simulink library "Tracked_ActiveSurveillance_Block"  (R2018b)
settings: Solver=VariableStepAuto  StartTime=0.0  StopTime=10.0  RelTol=1e-3
undefined symbols (not defined in the file): ac1dyn_alt0_ft, ac1dyn_lat0_rad, ac1dyn_lon0_rad, uas_tcas_dt_s, uas_tcas_trckd_altQuant_ft, uas_tcas_trckd_bearing_Breakpoints_deg, uas_tcas_trckd_bearing_Max_deg, uas_tcas_trckd_bearing_Sigma_deg, uas_tcas_trckd_FOR_elev_max_deg, uas_tcas_trckd_FOR_elev_min_deg, uas_tcas_trckd_probDetect, uas_tcas_trckd_psi_bias_rad, uas_tcas_trckd_psi_stddev_ft, uas_tcas_trckd_psidot_stddev_ftps, uas_tcas_trckd_randProbSeed, uas_tcas_trckd_reported_errorCovRBA, uas_tcas_trckd_rng_bias_ft, uas_tcas_trckd_rng_random_stddev_ft, uas_tcas_trckd_seed1, uas_tcas_trckd_seed2, uas_tcas_trckd_seed3, uas_tcas_trckd_seed4, uas_tcas_trckd_sns_max_front_range_ft, uas_tcas_trckd_sns_max_range_ft, uas_tcas_trckd_sns_max_rear_range_ft, uas_tcas_trckd_sns_max_side_range_ft, uas_tcas_trckd_tauThreshold_sec, uas_tcas_trckd_updateRate_sec
libraries: simulink x6, TSAA_Altitude_Error x1, dspmtrx3 x1
settings Model: Creator=BI28030  LastModifiedBy=BI28030

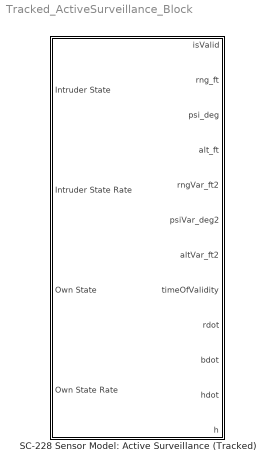
== system Tracked_ActiveSurveillance_Block ==
  SC-228 Sensor Model: Active Surveillance (Tracked) : Subsystem  mask(Tracked Surveillance: TCAS){dt_s=uas_tcas_dt_s, lat0_rad=ac1dyn_lat0_rad, lon0_rad=ac1dyn_lon0_rad, alt0_ft=ac1dyn_alt0_ft, sns_max_range_ft=uas_tcas_trckd_sns_max_range_ft, rng_random_stddev_ft=uas_tcas_trckd_rng_random_stddev_ft, rng_bias_ft=uas_tcas_trckd_rng_bias_ft, rng_tau_s=0, seed1=uas_tcas_trckd_seed1, bearing_Max_deg=uas_tcas_trckd_bearing_Max_deg, bearing_Sigma_deg=uas_tcas_trckd_bearing_Sigma_deg, bearing_Breakpoints_deg=uas_tcas_trckd_bearing_Breakpoints_deg, seed2=uas_tcas_trckd_seed2, seed3=uas_tcas_trckd_seed3, seed4=uas_tcas_trckd_seed4, altQuant_ft=uas_tcas_trckd_altQuant_ft, covRBA=uas_tcas_trckd_reported_errorCovRBA, sns_max_front_range_ft=uas_tcas_trckd_sns_max_front_range_ft, sns_max_side_range_ft=uas_tcas_trckd_sns_max_side_range_ft, sns_max_rear_range_ft=uas_tcas_trckd_sns_max_rear_range_ft, probDetect=uas_tcas_trckd_probDetect, FOR_elev_max_deg=uas_tcas_trckd_FOR_elev_max_deg, FOR_elev_min_deg=uas_tcas_trckd_FOR_elev_min_deg, randProbSeed=uas_tcas_trckd_randProbSeed, tauThreshold_sec=uas_tcas_trckd_tauThreshold_sec, updateRate_sec=uas_tcas_trckd_updateRate_sec}
      mask prompts: dt_s "Timestep (s)"; lat0_rad "ENU Reference Latitude (rad)"; lon0_rad "ENU Reference Longitude (rad)"; alt0_ft "ENU Reference Altitude (ft)"; sns_max_range_ft "Sensor Detection Range (ft)"; rng_random_stddev_ft "Random Error Standard Deviation (ft)"; rng_bias_ft "Bias Error (ft)"; rng_tau_s "Correlation Time (s)"; seed1 "Random Seed"; bearing_Max_deg "Bearing Max Error Table (deg)"; bearing_Sigma_deg "Bearing Sigma Table (deg)"; bearing_Breakpoints_deg "Bearing Breakpoints Table (deg)"; seed2 "Random Seed"; seed3 "Lambda Random Seed"; seed4 "Random Seed"; altQuant_ft "Altitude Quantization"; covRBA "Error Covariance Matrix"; sns_max_front_range_ft "Max Detection Range in Front (ft)"; sns_max_side_range_ft "Max Detection Range in Side (ft)"; sns_max_rear_range_ft "Max Detection Range in Back (ft)"; probDetect "Detection Probability"; FOR_elev_max_deg "Max FOR Elevation"; FOR_elev_min_deg "Min FOR Elevation"; randProbSeed "Random Seed"; tauThreshold_sec "Tau Threshold (Change Update Rates) seconds"; updateRate_sec "Update Rate (sec)"
      mask help: Additive noise model of TCAS with a tracker
      mask Help:
      | Additive noise model of TCAS. Independent noise is added to each
      | position and velocity component in a range-bearing-altitude coordinate
      | system.  Noise is colored using weights determined by time constant
      | parameters.
      | 
      | Output takes the form of a AircraftEstimate data bus and a 6x6 error covariance
      | matrix in North-East-Down.
      mask DialogControl ParameterTabVar0 Prompt: Tab
      mask DialogControl ParameterTabVar01 Prompt: Range
      mask DialogControl ParameterTabVar012 Prompt: Bearing
      mask DialogControl ParameterTabVar0123 Prompt: Altitude
      mask DialogControl ParameterTabVar0123456 Prompt: Covariance
      mask DialogControl ParameterTabVar01234567 Prompt: Detection

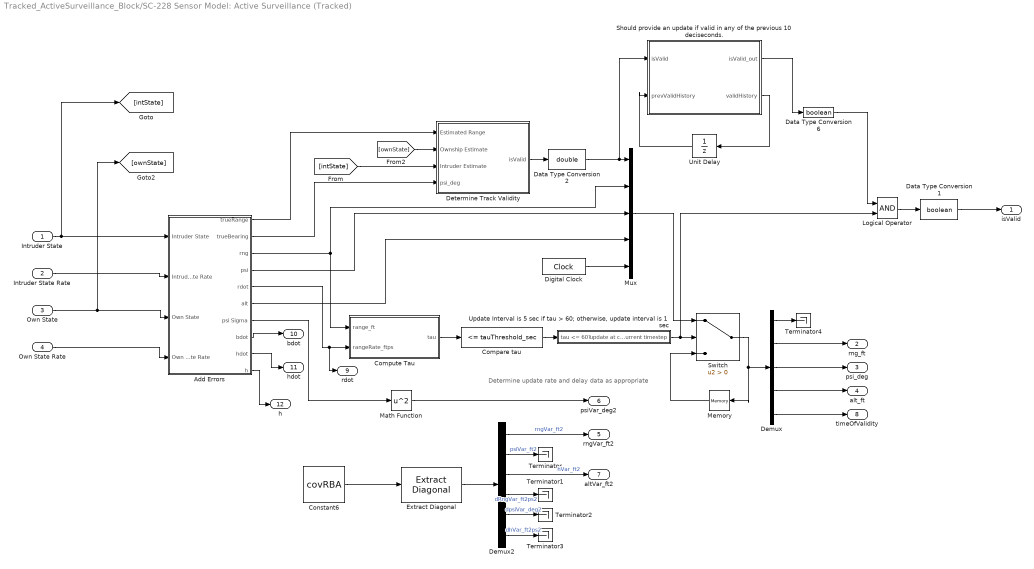
== system Tracked_ActiveSurveillance_Block/SC-228 Sensor Model: Active Surveillance (Tracked) ==
  note: Determine update rate and delay data as appropriate
  Intruder State : Inport  OutDataTypeStr=Bus: AircraftState
  Intruder State Rate : Inport  Port=2  OutDataTypeStr=Bus: AircraftStateRate
  Own State : Inport  Port=3  OutDataTypeStr=Bus: AircraftState
  Own State Rate : Inport  Port=4  OutDataTypeStr=Bus: AircraftStateRate
  Add Errors : Subsystem
  Compare tau : simulink/Logic and Bit Operations/Compare To Constant  relop=<=  const=tauThreshold_sec  OutDataTypeStr=boolean
  Compute Tau : Subsystem
  Constant6 : Constant  Value=covRBA
  Data Type Conversion1 : DataTypeConversion  OutDataTypeStr=boolean
  Data Type Conversion2 : DataTypeConversion  OutDataTypeStr=double
  Data Type Conversion6 : DataTypeConversion  OutDataTypeStr=boolean
  Demux : Demux  Outputs=5
  Demux2 : Demux  Outputs=6
  Determine Track Validity : Subsystem
  Digital Clock : DigitalClock  SampleTime=0.1
  Extract Diagonal : dspmtrx3/Extract Diagonal
      settings: SourceProductName=DSP System Toolbox  SourceProductBaseCode=DS
  Logical Operator : Logic  AllPortsSameDT=off  OutDataTypeStr=boolean
  Math Function : Math  Operator=square  SaturateOnIntegerOverflow=on
  Memory : Memory
  Mux : Mux  Inputs=5
  Should provide an update if valid in any of the previous 10 deciseconds. : MATLAB Function  TreatAsAtomicUnit=on
  Switch : Switch  Criteria=u2 > Threshold
  Terminator{,1..4} (5 alike) : Terminator
  Unit Delay : UnitDelay  SampleTime=-1
  "Update Interval is 5 sec if tau > 60; otherwise, update interval is 1 sec" : Subsystem  mask{updateRate=updateRate_sec}
      mask prompts: updateRate "Update Rate When Tau > 60"
  isValid : Outport
  rng_ft : Outport  Port=2
  psi_deg : Outport  Port=3
  alt_ft : Outport  Port=4
  rngVar_ft2 : Outport  Port=5
  psiVar_deg2 : Outport  Port=6
  altVar_ft2 : Outport  Port=7
  timeOfValidity : Outport  Port=8
  rdot : Outport  Port=9
  bdot : Outport  Port=10
  hdot : Outport  Port=11
  h : Outport  Port=12
  wires:
  Add Errors/4(psi) -> Mux/3
  Add Errors/10(h) -> h/1
  Add Errors/9(hdot) -> hdot/1
  Add Errors/8(bdot) -> bdot/1
  Unit Delay/1 -> Should provide an update if valid in any of the previous 10 deciseconds./2(prevValidHistory)
  Should provide an update if valid in any of the previous 10 deciseconds./2(validHistory) -> Unit Delay/1
  Data Type Conversion6/1 -> Logical Operator/1
  Data Type Conversion2/1 -> Mux/1, Should provide an update if valid in any of the previous 10 deciseconds./1(isValid)
  Should provide an update if valid in any of the previous 10 deciseconds./1(isValid_out) -> Data Type Conversion6/1
  "Update Interval is 5 sec if tau > 60; otherwise, update interval is 1 sec"/1(update at current timestep) -> Switch/2, Logical Operator/2
  Demux/1 -> Terminator4/1
  Math Function/1 -> psiVar_deg2/1
  Demux2/6 -> Terminator3/1  "dhVar_ft2ps2"
  Demux2/3 -> altVar_ft2/1  "hVar_ft2"
  Constant6/1 -> Extract Diagonal/1
  Demux2/1 -> rngVar_ft2/1  "rngVar_ft2"
  Demux2/2 -> Terminator/1  "psiVar_ft2"
  Demux2/5 -> Terminator2/1  "dpsiVar_deg2"
  Demux2/4 -> Terminator1/1  "dRngVar_ft2ps2"
  Extract Diagonal/1 -> Demux2/1
  Add Errors/7(psi Sigma) -> Math Function/1
  Data Type Conversion1/1 -> isValid/1
  Determine Track Validity/1(isValid) -> Data Type Conversion2/1
  Compare tau/1 -> "Update Interval is 5 sec if tau > 60; otherwise, update interval is 1 sec"/1(tau <= 60?)
  Memory/1 -> Switch/3
  Mux/1 -> Switch/1
  Demux/4 -> alt_ft/1
  Demux/3 -> psi_deg/1
  Demux/2 -> rng_ft/1
  Logical Operator/1 -> Data Type Conversion1/1
  Switch/1 -> Demux/1, Memory/1
  Compute Tau/1(tau) -> Compare tau/1
  Add Errors/5(rdot) -> Compute Tau/2(rangeRate_ftps), rdot/1
  Add Errors/6(alt) -> Mux/4
  [ownState] -> Determine Track Validity/2(Ownship Estimate)
  [intState] -> Determine Track Validity/3(Intruder Estimate)
  Own State Rate/1 -> Add Errors/4(Own State Rate)
  Add Errors/3(rng) -> Compute Tau/1(range_ft), Mux/2
  Own State/1 -> Add Errors/3(Own State), [ownState]
  Intruder State Rate/1 -> Add Errors/2(Intruder State Rate)
  Intruder State/1 -> Add Errors/1(Intruder State), [intState]
  Digital Clock/1 -> Mux/5
  Demux/5 -> timeOfValidity/1
  Add Errors/1(trueRange) -> Determine Track Validity/1(Estimated Range)
  Add Errors/2(trueBearing) -> Determine Track Validity/4(psi_deg)

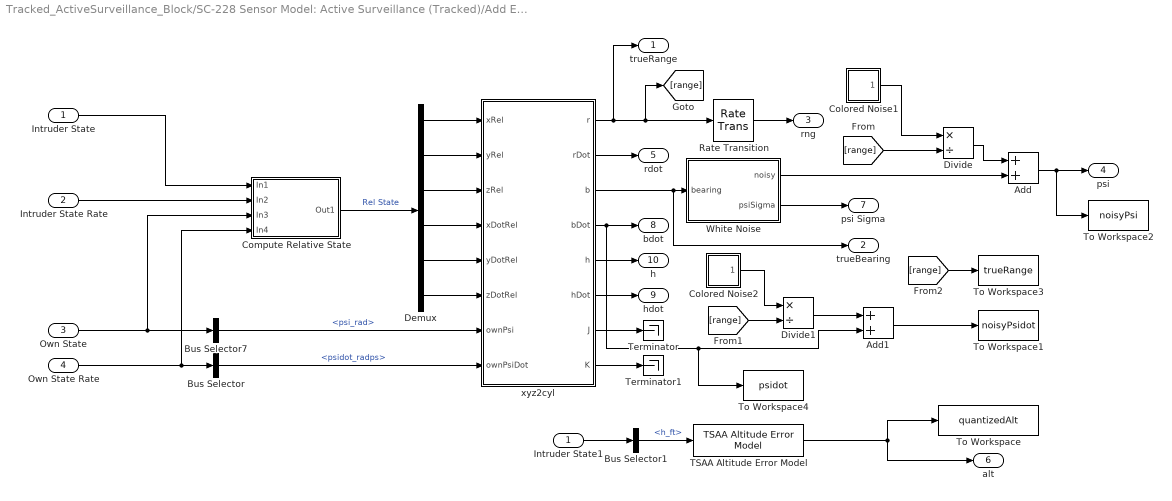
== system Tracked_ActiveSurveillance_Block/SC-228 Sensor Model: Active Surveillance (Tracked)/Add Errors ==
  Intruder State : Inport
  Intruder State Rate : Inport  Port=2  OutDataTypeStr=Bus: AircraftStateRate
  Own State : Inport  Port=3
  Own State Rate : Inport  Port=4
  Add : Sum
  Add1 : Sum
  Bus Selector : BusSelector  OutputSignals=psidot_radps
  Bus Selector1 : BusSelector  OutputSignals=h_ft
  Bus Selector7 : BusSelector  OutputSignals=psi_rad
  Colored Noise1 : Subsystem  mask(Colored Noise){sig=uas_tcas_trckd_psi_stddev_ft, bias=uas_tcas_trckd_psi_bias_rad, tau=0, dt=dt_s, seed=seed1}
      mask prompts: sig "Random error standard deviation"; bias "Bias error"; tau "Correlation time"; dt "Track update time"; seed "Random Seed"
      mask help: Generates a noisy state variable estimate using the ABSAA colored noise model. Set correlation time to zero for white noise.
      mask Help:
      | Generates a noisy state variable estimate using the AF Common ABSAA error
      | model.  Time correlation of the error is defined by an exponential decay
      | of K = exp(-tau/dt), where tau is the correlation time and dt is the time
      | between track updates.  The track error at time t is then:
      | 
      |     err(t) = K*err(t-1) + N(0,(1-K^2)*sig^2) + bias
      | 
      | where N(x,y) is a Gaussian noise process with mean x and variance y and
      | with random number generator seeded with the integer 'seed'.
      | 
      | The random noise process must be initialized with an error drawn from
      | N(0,sig^2).
      | 
      | The noise model can be used to produce white noise by setting tau to zero.
  Colored Noise2 : Subsystem  mask(Colored Noise){sig=uas_tcas_trckd_psidot_stddev_ftps, bias=uas_tcas_trckd_psi_bias_rad, tau=0, dt=dt_s, seed=seed2}
      mask prompts: sig "Random error standard deviation"; bias "Bias error"; tau "Correlation time"; dt "Track update time"; seed "Random Seed"
      mask help: Generates a noisy state variable estimate using the ABSAA colored noise model. Set correlation time to zero for white noise.
      mask Help:
      | Generates a noisy state variable estimate using the AF Common ABSAA error
      | model.  Time correlation of the error is defined by an exponential decay
      | of K = exp(-tau/dt), where tau is the correlation time and dt is the time
      | between track updates.  The track error at time t is then:
      | 
      |     err(t) = K*err(t-1) + N(0,(1-K^2)*sig^2) + bias
      | 
      | where N(x,y) is a Gaussian noise process with mean x and variance y and
      | with random number generator seeded with the integer 'seed'.
      | 
      | The random noise process must be initialized with an error drawn from
      | N(0,sig^2).
      | 
      | The noise model can be used to produce white noise by setting tau to zero.
  Compute Relative State : Subsystem
  Demux : Demux  Outputs=6
  Divide : Product  Inputs=*/
  Divide1 : Product  Inputs=*/
  Intruder State1 : InportShadow
  Rate Transition : RateTransition  OutPortSampleTime=0
  TSAA Altitude Error Model : TSAA_Altitude_Error/TSAA Altitude Error Model  ac_id=1  perfect=false  lambdaSeed=seed3  randomSeed=seed4  altQuant_ft=altQuant_ft  dt_s=0
  Terminator : Terminator
  Terminator1 : Terminator
  To Workspace : ToWorkspace  VariableName=quantizedAlt  SaveFormat=Timeseries  SampleTime=-1
  To Workspace1 : ToWorkspace  VariableName=noisyPsidot  SaveFormat=Timeseries  SampleTime=-1
  To Workspace2 : ToWorkspace  VariableName=noisyPsi  SaveFormat=Timeseries  SampleTime=-1
  To Workspace3 : ToWorkspace  VariableName=trueRange  SaveFormat=Timeseries  SampleTime=-1
  To Workspace4 : ToWorkspace  VariableName=psidot  SaveFormat=Timeseries  SampleTime=-1
  White Noise : Subsystem  mask{bearing_Max_deg=bearing_Max_deg, bearing_Sigma_deg=bearing_Sigma_deg, bearing_Breakpoints_deg=bearing_Breakpoints_deg, seed_bearing=seed2}
      mask prompts: bearing_Max_deg "Bearing Max Error Table (deg)"; bearing_Sigma_deg "Bearing Sigma Table (deg)"; bearing_Breakpoints_deg "Bearing Breakpoints Table (deg)"; seed_bearing "Random Seed"
  xyz2cyl : MATLAB Function  TreatAsAtomicUnit=on
  trueRange : Outport
  trueBearing : Outport  Port=2
  rng : Outport  Port=3
  psi : Outport  Port=4
  rdot : Outport  Port=5
  alt : Outport  Port=6
  psi Sigma : Outport  Port=7
  bdot : Outport  Port=8
  hdot : Outport  Port=9
  h : Outport  Port=10
  wires:
  [range] -> To Workspace3/1
  Add1/1 -> To Workspace1/1
  [range] -> Divide1/2
  [range] -> Divide/2
  Divide1/1 -> Add1/1
  Colored Noise2/1(noisy) -> Divide1/1
  Add/1 -> psi/1, To Workspace2/1
  Divide/1 -> Add/1
  Colored Noise1/1(noisy) -> Divide/1
  Intruder State1/1 -> Bus Selector1/1
  TSAA Altitude Error Model/1 -> alt/1, To Workspace/1
  White Noise/2(psiSigma) -> psi Sigma/1
  White Noise/1("noisy ") -> Add/2
  xyz2cyl/3(b) -> White Noise/1(bearing), trueBearing/1
  xyz2cyl/6(hDot) -> hdot/1
  xyz2cyl/4(bDot) -> bdot/1, Add1/2, To Workspace4/1
  xyz2cyl/2(rDot) -> rdot/1
  xyz2cyl/8(K) -> Terminator1/1
  xyz2cyl/7(J) -> Terminator/1
  Bus Selector/1 -> xyz2cyl/8(ownPsiDot)  "<psidot_radps>"
  Own State Rate/1 -> Bus Selector/1, Compute Relative State/4(In4)
  Demux/4 -> xyz2cyl/4(xDotRel)
  Demux/2 -> xyz2cyl/2(yRel)
  xyz2cyl/5(h) -> h/1
  xyz2cyl/1(r) -> [range], Rate Transition/1, trueRange/1
  Demux/3 -> xyz2cyl/3(zRel)
  Demux/1 -> xyz2cyl/1(xRel)
  Compute Relative State/1(Out1) -> Demux/1  "Rel State"
  Demux/6 -> xyz2cyl/6(zDotRel)
  Bus Selector7/1 -> xyz2cyl/7(ownPsi)  "<psi_rad>"
  Intruder State Rate/1 -> Compute Relative State/2(In2)
  Own State/1 -> Compute Relative State/3(In3), Bus Selector7/1
  Intruder State/1 -> Compute Relative State/1(In1)
  Demux/5 -> xyz2cyl/5(yDotRel)
  Bus Selector1/1 -> TSAA Altitude Error Model/1  "<h_ft>"
  Rate Transition/1 -> rng/1

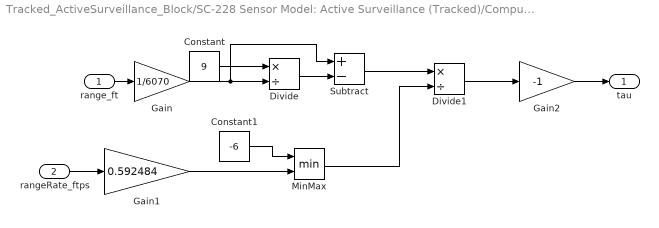
== system Tracked_ActiveSurveillance_Block/SC-228 Sensor Model: Active Surveillance (Tracked)/Compute Tau ==
  range_ft : Inport
  rangeRate_ftps : Inport  Port=2
  Constant : Constant  Value=9
  Constant1 : Constant  Value=-6
  Divide : Product  Inputs=*/
  Divide1 : Product  Inputs=*/
  Gain : Gain  Gain=1/6070
  Gain1 : Gain  Gain=0.592484
  Gain2 : Gain  Gain=-1
  MinMax : MinMax  Inputs=2
  Subtract : Sum  Inputs=+-
  tau : Outport
  wires:
  Gain2/1 -> tau/1
  MinMax/1 -> Divide1/2
  Constant1/1 -> MinMax/1
  Gain1/1 -> MinMax/2
  Subtract/1 -> Divide1/1
  Divide/1 -> Subtract/2
  Constant/1 -> Divide/1
  Gain/1 -> Divide/2, Subtract/1
  range_ft/1 -> Gain/1
  Divide1/1 -> Gain2/1
  rangeRate_ftps/1 -> Gain1/1

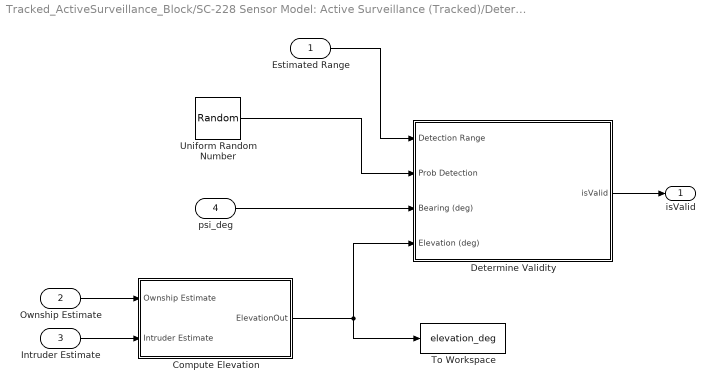
== system Tracked_ActiveSurveillance_Block/SC-228 Sensor Model: Active Surveillance (Tracked)/Determine Track Validity ==
  Estimated Range : Inport
  Ownship Estimate : Inport  Port=2
  Intruder Estimate : Inport  Port=3
  psi_deg : Inport  Port=4
  Compute Elevation : Subsystem
  "Determine Validity " : Subsystem  mask{sns_max_front_range_ft=sns_max_front_range_ft, sns_max_side_range_ft=sns_max_side_range_ft, sns_max_rear_range_ft=sns_max_rear_range_ft, FOR_elev_min_deg=FOR_elev_min_deg, FOR_elev_max_deg=FOR_elev_max_deg, probDetect=probDetect}
      mask prompts: sns_max_front_range_ft "Max Front Detection Range (ft)"; sns_max_side_range_ft "Max Side Detection Range (ft)"; sns_max_rear_range_ft "Max Rear Detection Range (ft)"; FOR_elev_min_deg "Min Elevation FOR (deg)"; FOR_elev_max_deg "Max Elevation FOR (deg)"; probDetect "Probability of Detection"
  To Workspace : ToWorkspace  VariableName=elevation_deg  SaveFormat=Timeseries  SampleTime=-1
  Uniform Random Number : UniformRandomNumber  Minimum=0  Seed=randProbSeed  SampleTime=dt_s
  isValid : Outport
  wires:
  psi_deg/1 -> "Determine Validity "/3(Bearing (deg))
  Intruder Estimate/1 -> Compute Elevation/2(Intruder Estimate)
  Compute Elevation/1(ElevationOut) -> To Workspace/1, "Determine Validity "/4(Elevation (deg))
  Ownship Estimate/1 -> Compute Elevation/1(Ownship Estimate)
  "Determine Validity "/1(isValid) -> isValid/1
  Uniform Random Number/1 -> "Determine Validity "/2(Prob Detection)
  Estimated Range/1 -> "Determine Validity "/1(Detection Range)

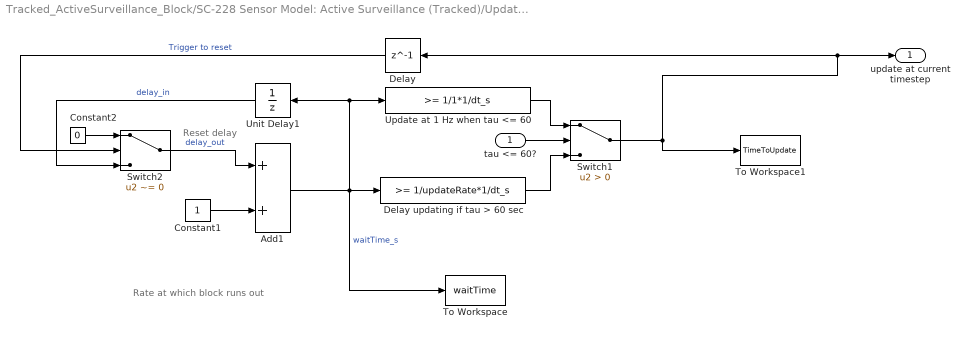
== system Tracked_ActiveSurveillance_Block/SC-228 Sensor Model: Active Surveillance (Tracked)/Update Interval is 5 sec if tau > 60; otherwise, update interval is 1 sec ==
  note: Rate at which block runs out
  note: Reset delay
  tau <= 60? : Inport
  Add1 : Sum
  Constant1 : Constant
  Constant2 : Constant  Value=0
  Delay : Delay  DelayLength=1  InitialCondition=0
  Delay updating if tau > 60 sec : simulink/Logic and Bit Operations/Compare To Constant  relop=>=  const=1/updateRate*1/dt_s  OutDataTypeStr=boolean
  Switch1 : Switch  Criteria=u2 > Threshold
  Switch2 : Switch  Criteria=u2 ~= 0  Threshold=true
  To Workspace : ToWorkspace  VariableName=waitTime  SaveFormat=Timeseries  SampleTime=-1
  To Workspace1 : ToWorkspace  VariableName=TimeToUpdate  SaveFormat=Timeseries  SampleTime=-1
  Unit Delay1 : UnitDelay  InitialCondition=-1  SampleTime=-1
  Update at 1 Hz when tau <= 60 : simulink/Logic and Bit Operations/Compare To Constant  relop=>=  const=1/1*1/dt_s  OutDataTypeStr=boolean
  update at current timestep : Outport
  wires:
  Switch1/1 -> To Workspace1/1, Delay/1, update at current timestep/1
  Switch2/1 -> Add1/1  "delay_out"
  Constant2/1 -> Switch2/1
  Unit Delay1/1 -> Switch2/3  "delay_in"
  Constant1/1 -> Add1/2
  Add1/1 -> Delay updating if tau > 60 sec/1, To Workspace/1, Update at 1 Hz when tau <= 60/1, Unit Delay1/1  "waitTime_s"
  Delay/1 -> Switch2/2  "Trigger to reset"
  tau <= 60?/1 -> Switch1/2
  Delay updating if tau > 60 sec/1 -> Switch1/3
  Update at 1 Hz when tau <= 60/1 -> Switch1/1

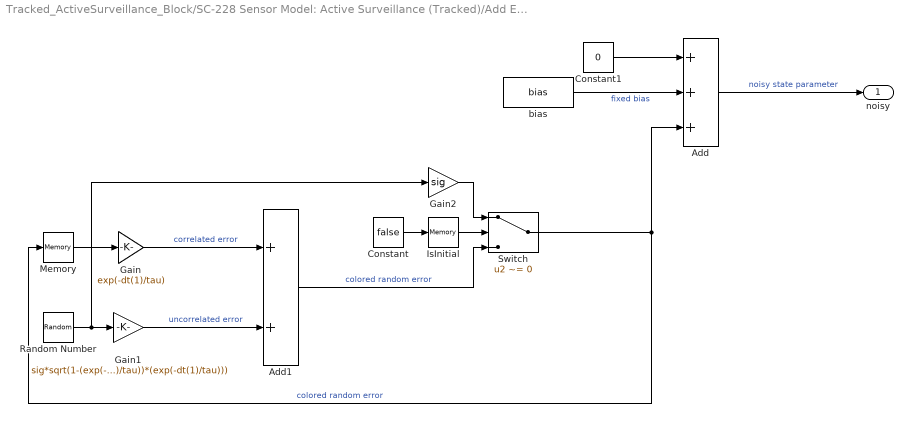
== system Tracked_ActiveSurveillance_Block/SC-228 Sensor Model: Active Surveillance (Tracked)/Add Errors/Colored Noise1 ==
  Add : Sum  Inputs=+++
  Add1 : Sum
  Constant : Constant  Value=false
  Constant1 : Constant  Value=0
  Gain : Gain  Gain=exp(-dt(1)/tau)
  Gain1 : Gain  Gain=sig*sqrt(1-(exp(-dt(1)/tau))*(exp(-dt(1)/tau)))
  Gain2 : Gain  Gain=sig
  IsInitial : Memory  InitialCondition=true  InheritSampleTime=on
  Memory : Memory  InheritSampleTime=on
  Random Number : RandomNumber  Seed=seed  SampleTime=dt_s
  Switch : Switch  Criteria=u2 ~= 0
  bias : Constant  Value=bias
  noisy : Outport
  wires:
  Constant1/1 -> Add/1
  Gain2/1 -> Switch/1
  Add1/1 -> Switch/3  "colored random error"
  IsInitial/1 -> Switch/2
  Constant/1 -> IsInitial/1
  Memory/1 -> Gain/1
  Add/1 -> noisy/1  "noisy state parameter"
  Gain/1 -> Add1/1  "correlated error"
  Random Number/1 -> Gain1/1, Gain2/1
  bias/1 -> Add/2  "fixed bias"
  Switch/1 -> Add/3, Memory/1  "colored random error"
  Gain1/1 -> Add1/2  "uncorrelated error"

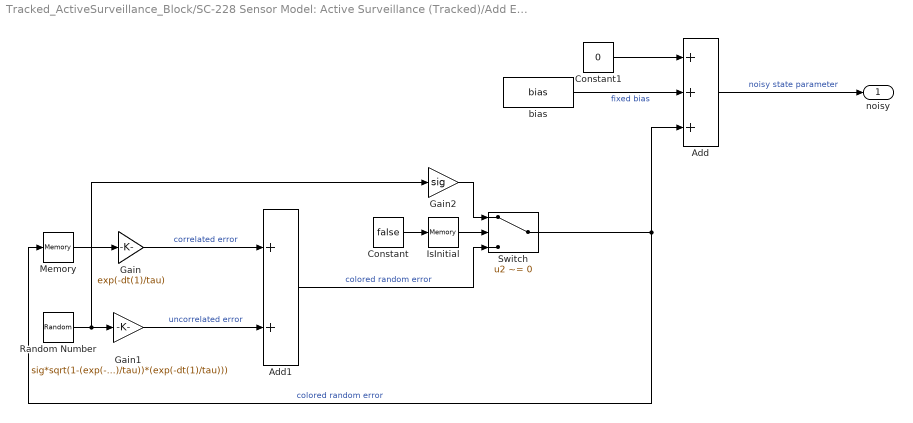
== system Tracked_ActiveSurveillance_Block/SC-228 Sensor Model: Active Surveillance (Tracked)/Add Errors/Colored Noise2 ==
  Add : Sum  Inputs=+++
  Add1 : Sum
  Constant : Constant  Value=false
  Constant1 : Constant  Value=0
  Gain : Gain  Gain=exp(-dt(1)/tau)
  Gain1 : Gain  Gain=sig*sqrt(1-(exp(-dt(1)/tau))*(exp(-dt(1)/tau)))
  Gain2 : Gain  Gain=sig
  IsInitial : Memory  InitialCondition=true  InheritSampleTime=on
  Memory : Memory  InheritSampleTime=on
  Random Number : RandomNumber  Seed=seed  SampleTime=dt_s
  Switch : Switch  Criteria=u2 ~= 0
  bias : Constant  Value=bias
  noisy : Outport
  wires:
  Constant1/1 -> Add/1
  Gain2/1 -> Switch/1
  Add1/1 -> Switch/3  "colored random error"
  IsInitial/1 -> Switch/2
  Constant/1 -> IsInitial/1
  Memory/1 -> Gain/1
  Add/1 -> noisy/1  "noisy state parameter"
  Gain/1 -> Add1/1  "correlated error"
  Random Number/1 -> Gain1/1, Gain2/1
  bias/1 -> Add/2  "fixed bias"
  Switch/1 -> Add/3, Memory/1  "colored random error"
  Gain1/1 -> Add1/2  "uncorrelated error"

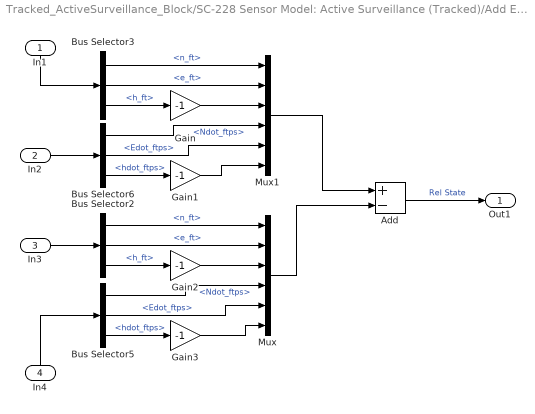
== system Tracked_ActiveSurveillance_Block/SC-228 Sensor Model: Active Surveillance (Tracked)/Add Errors/Compute Relative State ==
  In1 : Inport
  In2 : Inport  Port=2
  In3 : Inport  Port=3
  In4 : Inport  Port=4
  Add : Sum  Inputs=+-
  Bus Selector2 : BusSelector  OutputSignals=n_ft,e_ft,h_ft
  Bus Selector3 : BusSelector  OutputSignals=n_ft,e_ft,h_ft
  Bus Selector5 : BusSelector  OutputSignals=Ndot_ftps,Edot_ftps,hdot_ftps
  Bus Selector6 : BusSelector  OutputSignals=Ndot_ftps,Edot_ftps,hdot_ftps
  Gain{,1..3} (4 alike) : Gain  Gain=-1
  Mux : Mux  Inputs=6
  Mux1 : Mux  Inputs=6
  Out1 : Outport
  wires:
  Gain3/1 -> Mux/6
  Gain2/1 -> Mux/3
  Gain1/1 -> Mux1/6
  Gain/1 -> Mux1/3
  Bus Selector6/2 -> Mux1/5  "<Edot_ftps>"
  Bus Selector6/1 -> Mux1/4  "<Ndot_ftps>"
  Bus Selector6/3 -> Gain1/1  "<hdot_ftps>"
  In1/1 -> Bus Selector3/1
  Bus Selector3/2 -> Mux1/2  "<e_ft>"
  Bus Selector3/1 -> Mux1/1  "<n_ft>"
  Bus Selector2/1 -> Mux/1  "<n_ft>"
  Mux/1 -> Add/2
  Add/1 -> Out1/1  "Rel State"
  In3/1 -> Bus Selector2/1
  In4/1 -> Bus Selector5/1
  Mux1/1 -> Add/1
  Bus Selector2/2 -> Mux/2  "<e_ft>"
  Bus Selector5/3 -> Gain3/1  "<hdot_ftps>"
  Bus Selector2/3 -> Gain2/1  "<h_ft>"
  Bus Selector3/3 -> Gain/1  "<h_ft>"
  In2/1 -> Bus Selector6/1
  Bus Selector5/2 -> Mux/5  "<Edot_ftps>"
  Bus Selector5/1 -> Mux/4  "<Ndot_ftps>"

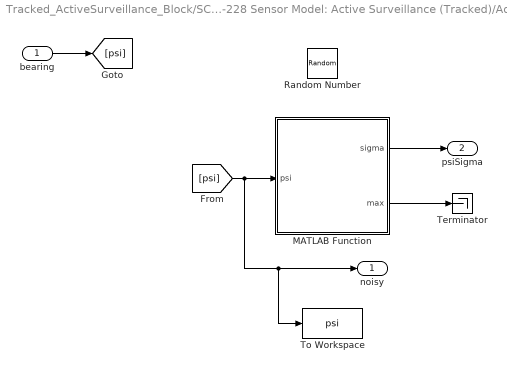
== system Tracked_ActiveSurveillance_Block/SC-228 Sensor Model: Active Surveillance (Tracked)/Add Errors/White Noise ==
  bearing : Inport
  MATLAB Function : MATLAB Function  TreatAsAtomicUnit=on
  Random Number : RandomNumber  Seed=seed_bearing  SampleTime=dt_s
  Terminator : Terminator
  To Workspace : ToWorkspace  VariableName=psi  SaveFormat=Timeseries  SampleTime=-1
  "noisy " : Outport
  psiSigma : Outport  Port=2
  wires:
  [psi] -> MATLAB Function/1(psi), "noisy "/1, To Workspace/1
  bearing/1 -> [psi]
  MATLAB Function/2(max) -> Terminator/1
  MATLAB Function/1(sigma) -> psiSigma/1

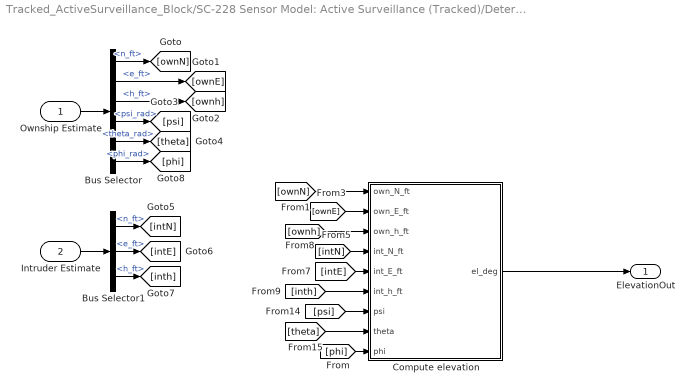
== system Tracked_ActiveSurveillance_Block/SC-228 Sensor Model: Active Surveillance (Tracked)/Determine Track Validity/Compute Elevation ==
  Ownship Estimate : Inport
  Intruder Estimate : Inport  Port=2
  Bus Selector : BusSelector  OutputSignals=n_ft,e_ft,h_ft,psi_rad,theta_rad,phi_rad
  Bus Selector1 : BusSelector  OutputSignals=n_ft,e_ft,h_ft
  Compute elevation : MATLAB Function  TreatAsAtomicUnit=on
  ElevationOut : Outport
  wires:
  [phi] -> Compute elevation/9(phi)
  Bus Selector/6 -> [phi]  "<phi_rad>"
  [theta] -> Compute elevation/8(theta)
  [psi] -> Compute elevation/7(psi)
  [inth] -> Compute elevation/6(int_h_ft)
  [ownh] -> Compute elevation/3(own_h_ft)
  [intE] -> Compute elevation/5(int_E_ft)
  [intN] -> Compute elevation/4(int_N_ft)
  [ownE] -> Compute elevation/2(own_E_ft)
  [ownN] -> Compute elevation/1(own_N_ft)
  Bus Selector1/3 -> [inth]  "<h_ft>"
  Bus Selector1/2 -> [intE]  "<e_ft>"
  Bus Selector1/1 -> [intN]  "<n_ft>"
  Bus Selector/5 -> [theta]  "<theta_rad>"
  Bus Selector/4 -> [psi]  "<psi_rad>"
  Bus Selector/3 -> [ownh]  "<h_ft>"
  Bus Selector/2 -> [ownE]  "<e_ft>"
  Bus Selector/1 -> [ownN]  "<n_ft>"
  Intruder Estimate/1 -> Bus Selector1/1
  Compute elevation/1(el_deg) -> ElevationOut/1
  Ownship Estimate/1 -> Bus Selector/1

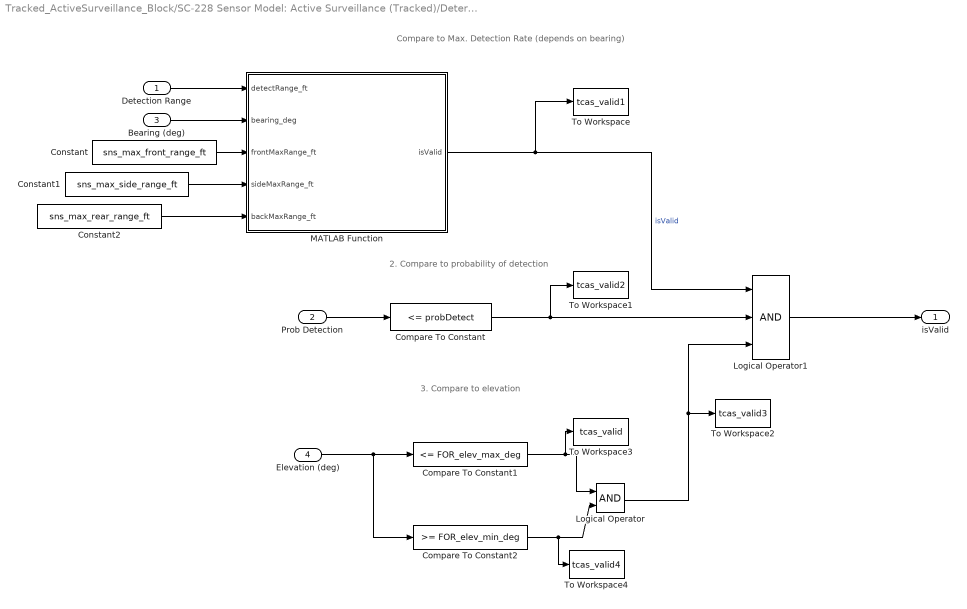
== system Tracked_ActiveSurveillance_Block/SC-228 Sensor Model: Active Surveillance (Tracked)/Determine Track Validity/Determine Validity  ==
  note: Compare to Max. Detection Rate (depends on bearing)
  note: 2. Compare to probability of detection
  note: 3. Compare to elevation
  Detection Range : Inport
  Prob Detection : Inport  Port=2
  Bearing (deg) : Inport  Port=3
  Elevation (deg) : Inport  Port=4
  Compare To Constant : simulink/Logic and Bit Operations/Compare To Constant  relop=<=  const=probDetect  OutDataTypeStr=boolean
  Compare To Constant1 : simulink/Logic and Bit Operations/Compare To Constant  relop=<=  const=FOR_elev_max_deg  OutDataTypeStr=boolean
  Compare To Constant2 : simulink/Logic and Bit Operations/Compare To Constant  relop=>=  const=FOR_elev_min_deg  OutDataTypeStr=boolean
  Constant : Constant  Value=sns_max_front_range_ft
  Constant1 : Constant  Value=sns_max_side_range_ft
  Constant2 : Constant  Value=sns_max_rear_range_ft
  Logical Operator : Logic  AllPortsSameDT=off  OutDataTypeStr=boolean
  Logical Operator1 : Logic  Inputs=3  AllPortsSameDT=off  OutDataTypeStr=boolean
  MATLAB Function : MATLAB Function  TreatAsAtomicUnit=on
  To Workspace : ToWorkspace  VariableName=tcas_valid1  SaveFormat=Timeseries  SampleTime=-1
  To Workspace1 : ToWorkspace  VariableName=tcas_valid2  SaveFormat=Timeseries  SampleTime=-1
  To Workspace2 : ToWorkspace  VariableName=tcas_valid3  SaveFormat=Timeseries  SampleTime=-1
  To Workspace3 : ToWorkspace  VariableName=tcas_valid  SaveFormat=Timeseries  SampleTime=-1
  To Workspace4 : ToWorkspace  VariableName=tcas_valid4  SaveFormat=Timeseries  SampleTime=-1
  isValid : Outport
  wires:
  Constant2/1 -> MATLAB Function/5(backMaxRange_ft)
  Constant1/1 -> MATLAB Function/4(sideMaxRange_ft)
  Constant/1 -> MATLAB Function/3(frontMaxRange_ft)
  Bearing (deg)/1 -> MATLAB Function/2(bearing_deg)
  Logical Operator/1 -> To Workspace2/1, Logical Operator1/3
  Logical Operator1/1 -> isValid/1
  Compare To Constant2/1 -> To Workspace4/1, Logical Operator/2
  Compare To Constant1/1 -> To Workspace3/1, Logical Operator/1
  Elevation (deg)/1 -> Compare To Constant1/1, Compare To Constant2/1
  Compare To Constant/1 -> To Workspace1/1, Logical Operator1/2
  Prob Detection/1 -> Compare To Constant/1
  MATLAB Function/1(isValid) -> To Workspace/1, Logical Operator1/1  "isValid"
  Detection Range/1 -> MATLAB Function/1(detectRange_ft)

== matlab function Tracked_ActiveSurveillance_Block/SC-228 Sensor Model: Active Surveillance (Tracked)/Add Errors/White Noise/MATLAB Function ==
  data: psi input; sigma output; max output
function [sigma, max]= fcn(psi)
%#codegen
sigma = 0; max = 0;

bearing_Breakpoints_deg = [-9999, -15, -10, 10, 20, 9999]';
bearing_Sigma_deg = [15, 15, 15, 9, 15, 15];
bearing_Max_deg = [45, 45, 45, 27, 45, 45];

index = find(psi<bearing_Breakpoints_deg,1);
index = index(1);

sigma = bearing_Sigma_deg(index);
max = bearing_Max_deg(index);

== matlab function Tracked_ActiveSurveillance_Block/SC-228 Sensor Model: Active Surveillance (Tracked)/Add Errors/xyz2cyl ==
  data: xRel input; r output; yRel input; zRel input; xDotRel input; yDotRel input; zDotRel input; ownPsi input; ownPsiDot input; rDot output; b output; bDot output; h output; hDot output; J output; K output
function [r,rDot,b,bDot,h,hDot,J,K] = fcn(xRel,yRel,zRel,xDotRel,yDotRel,zDotRel,ownPsi,ownPsiDot)
%#codegen
% Convert position and velocity of intruder relative to ownship from 
% Cartesian coordinates in North-East-Down system to range/bearing/altitude
% coordinates.  Also returns Jacobian blocks J and K, where 6x6 Jacobian =
% [J zeros; K J]

r = norm([xRel yRel zRel]);
h = -zRel;
b = atan2(yRel,xRel) - ownPsi;

rDot = dot([xRel yRel zRel], [xDotRel yDotRel zDotRel])/r;
hDot = -zDotRel;
bDot = (yDotRel*xRel - yRel*xDotRel)/(xRel^2 + yRel^2) - ownPsiDot;

r2D = norm([xRel yRel]);

% Jacobian elements

J = [  xRel/r   yRel/r   zRel/r ;
     -yRel/r2D^2 xRel/r2D^2    0    ;
          0       0       -1   ];
      
K = zeros(3,3);
K(1,1) = xDotRel/r - xRel*rDot/r^2;
K(1,2) = yDotRel/r - yRel*rDot/r^2;
K(1,3) = zDotRel/r - zRel*rDot/r^2;
K(2,1) = (yDotRel*yRel^2 + 2*xRel*xDotRel*yRel - yDotRel*xRel^2)/r2D^4;
K(2,2) = (xDotRel*yRel^2 - 2*xRel*yRel*yDotRel - xRel^2*xDotRel)/r2D^4;

b = b*180/pi;

== matlab function Tracked_ActiveSurveillance_Block/SC-228 Sensor Model: Active Surveillance (Tracked)/Determine Track Validity/Compute Elevation/Compute elevation ==
  data: own_N_ft input; el_deg output; own_E_ft input; own_h_ft input; int_N_ft input; int_E_ft input; int_h_ft input; psi input; theta input; phi input
function el_deg = fcn(own_N_ft, own_E_ft, own_h_ft, int_N_ft, int_E_ft, int_h_ft, psi, theta, phi)
%#codegen
Ri = [int_N_ft-own_N_ft; int_E_ft-own_E_ft; -(int_h_ft-own_h_ft)];

ct   = cos(-theta);
st   = sin(-theta);
cphi = cos(phi); %1;%
sphi = sin(phi); %0;%
cpsi = cos(psi);
spsi = sin(psi);

M = [ ct*cpsi                  ct*spsi                     -st; ...
      sphi*st*cpsi-cphi*spsi   sphi*st*spsi+cphi*cpsi      sphi*ct; ...
      cphi*st*cpsi+sphi*spsi   cphi*st*spsi-sphi*cpsi      cphi*ct ];
  
Rb = M*Ri;

R = sqrt( Ri(1)^2+Ri(2)^2+Ri(3)^2 );
el = asin( Rb(3)/R );
el_deg = el*180/pi;

% roll = phi_deg;
% pitch = theta_deg;
% heading = psi_deg;
% 
% Ri = [int_N_ft-own_N_ft; int_E_ft-own_E_ft; -(int_h_ft-own_h_ft)];
% 
% Mroll = [1, 0, 0;...
%     0, cos(roll), sin(roll);...
%     0, -sin(roll), cos(roll)];
% 
% Mpitch = [cos(pitch), 0, -sin(pitch);...
%     0, 1, 0;...
%     sin(pitch), 0, cos(pitch)];
% 
% Mhead = [cos(heading), sin(heading), 0;...
%     -sin(heading), cos(heading), 0;...
%     0, 0, 1];
% 
% Mi2b = Mroll*Mpitch*Mhead; % inertial to body
%   
% Rb = Mi2b*Ri;
% 
% %R = sqrt( Ri(1)^2+Ri(2)^2+Ri(3)^2 );
% %az = atan2( Rb(2), Rb(1) );
% el = atan( -Rb(3)/sqrt(Ri(1)^2+Ri(2)^2) );
% 
% el_deg = el*180/pi;

end

== matlab function Tracked_ActiveSurveillance_Block/SC-228 Sensor Model: Active Surveillance (Tracked)/Determine Track Validity/Determine Validity /MATLAB Function ==
  data: detectRange_ft input; isValid output; bearing_deg input; frontMaxRange_ft input; sideMaxRange_ft input; backMaxRange_ft input
function isValid = fcn(detectRange_ft, bearing_deg, frontMaxRange_ft, sideMaxRange_ft, backMaxRange_ft)
isValid = false;

%Need to wrap bearing_deg to 180
if bearing_deg >=180
    bearing_deg = bearing_deg - 2*180;
elseif bearing_deg <-180
    bearing_deg = bearing_deg + 2*180;
end

%#codegen
if(bearing_deg>=-45 && bearing_deg <=45) %front
    isValid = detectRange_ft<frontMaxRange_ft;
    
elseif (bearing_deg>=-135 && bearing_deg <=-45) || (bearing_deg>=45 && bearing_deg <=135) %side
    isValid = detectRange_ft<sideMaxRange_ft;
    
elseif (bearing_deg>=-180 && bearing_deg <=-135) || (bearing_deg>=135 && bearing_deg <=180) %back
    isValid = detectRange_ft<backMaxRange_ft;
    
end

== matlab function Tracked_ActiveSurveillance_Block/SC-228 Sensor Model: Active Surveillance (Tracked)/Should provide an update if valid in any of the previous 10 deciseconds. ==
  settings: updateMethod=DISCRETE  sampleTime=dt_s
  data: isValid_out output; isValid input; prevValidHistory input; validHistory output
function [isValid_out, validHistory] = determineValidity(isValid, prevValidHistory)
%#codegen
validHistory = [isValid, prevValidHistory(1:9)];

isValid_out = max(validHistory);
